simulink model "Multiagent_1030_ActorCritic"  (R2023a)
settings: Solver=FixedStepAuto  StartTime=0.0  StopTime=500  FixedStep=0.001  RelTol=1e-3
values from neighbouring files (symbols this model uses):
  INT_1 = [0;0.5;0]    [Paramaters.m]
  INT_2 = [-3.5;6;0]    [Paramaters.m]
  INT_3 = [-7.1;10;0.0]    [Paramaters.m]
  INT_4 = [-10.5;15;0.2]    [Paramaters.m]
  INT_5 = [-14;20;0.4]    [Paramaters.m]
(part 1 of 2)
settings Model: Creator=Admin  LastModifiedBy=ADMIN
settings DataIOCC: ReturnWorkspaceOutputs=off
settings DebuggingCC: UnconnectedInputMsg=warning  UnconnectedOutputMsg=warning  UnconnectedLineMsg=warning
settings ModelReferenceCC: EnableRefExpFcnMdlSchedulingChecks=on
settings RTWCC: DLArmComputeVersion=19.05

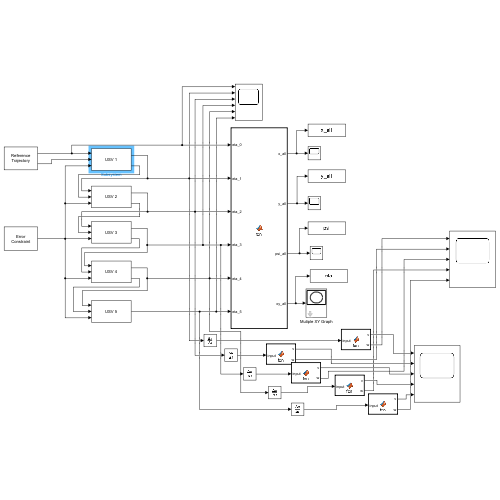
[thumbnail: Simulink's stored preview of the top-level diagram]
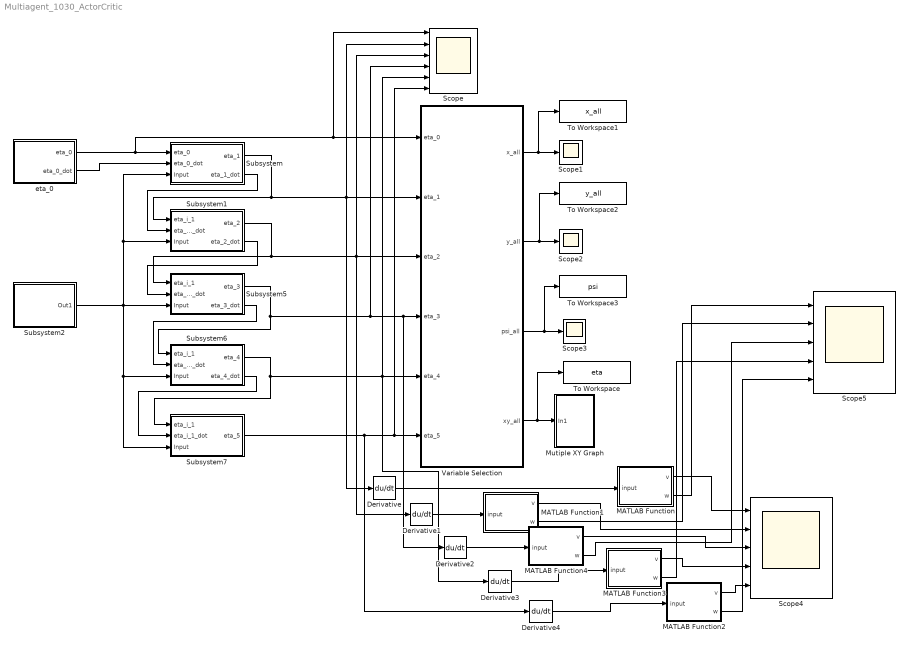
== system Multiagent_1030_ActorCritic ==
  Derivative{,1..4} (5 alike) : Derivative
  MATLAB Function : MATLAB Function  TreatAsAtomicUnit=on
  MATLAB Function1 : MATLAB Function  TreatAsAtomicUnit=on
  MATLAB Function2 : MATLAB Function  TreatAsAtomicUnit=on
  MATLAB Function3 : MATLAB Function  TreatAsAtomicUnit=on
  MATLAB Function4 : MATLAB Function  TreatAsAtomicUnit=on
  Mutiple XY Graph : Subsystem  mask(Mutiple XY Graph){number_of_trajectories=5, axis_limits=[-40 80 -10 110], sample_time=1}
      mask prompts: number_of_trajectories "Number of Trajectories"; axis_limits "Axis Limits"; sample_time "Sample Time"
      mask Display: plot([.05 .95 .95 .05 .05],[.45 .45 .95 .95 .45], 0.5+cos(0:0.1:2*pi)*0.3,0.7+sin(0:0.1:2*pi)*0.2)
  Scope : Scope  NumInputPorts=6
  Scope1 : Scope
  Scope2 : Scope
  Scope3 : Scope
  Scope4 : Scope  NumInputPorts=5
  Scope5 : Scope  NumInputPorts=5
  Subsystem : Subsystem
      mask Display: disp('USV 1')
  Subsystem1 : Subsystem
      mask Display: disp('USV 2')
  Subsystem2 : Subsystem
      mask Display: disp('Error\nConstraint');
  Subsystem5 : Subsystem
      mask Display: disp('USV 3')
  Subsystem6 : Subsystem
      mask Display: disp('USV 4')
  Subsystem7 : Subsystem
      mask Display: disp('USV 5')
  To Workspace : ToWorkspace  VariableName=eta  SaveFormat=Timeseries  SampleTime=-1
  To Workspace1 : ToWorkspace  VariableName=x_all  SaveFormat=Timeseries  SampleTime=-1
  To Workspace2 : ToWorkspace  VariableName=y_all  SaveFormat=Timeseries  SampleTime=-1
  To Workspace3 : ToWorkspace  VariableName=psi  SaveFormat=Timeseries  SampleTime=-1
  Variable Selection : MATLAB Function  TreatAsAtomicUnit=on
  eta_0 : Subsystem
      mask Display: disp('Reference\nTrajectory')
  wires:
  Subsystem/1(eta_1) -> Subsystem1/1(eta_i_1), Scope/2, Variable Selection/2(eta_1), Derivative/1
  Variable Selection/4(xy_all) -> To Workspace/1, Mutiple XY Graph/1(In1)
  eta_0/1(eta_0) -> Scope/1, Variable Selection/1(eta_0), Subsystem/1(eta_0)
  eta_0/2(eta_0_dot) -> Subsystem/2(eta_0_dot)
  Subsystem/2(eta_1_dot) -> Subsystem1/2(eta_i_1_dot)
  Subsystem1/1(eta_2) -> Variable Selection/3(eta_2), Scope/3, Derivative1/1, Subsystem5/1(eta_i_1)
  Variable Selection/1(x_all) -> To Workspace1/1, Scope1/1
  Variable Selection/2(y_all) -> To Workspace2/1, Scope2/1
  Variable Selection/3(psi_all) -> To Workspace3/1, Scope3/1
  Subsystem7/1(eta_5) -> Variable Selection/6(eta_5), Scope/6, Derivative4/1
  Subsystem6/1(eta_4) -> Subsystem7/1(eta_i_1), Scope/5, Variable Selection/5(eta_4), Derivative3/1
  Subsystem6/2(eta_4_dot) -> Subsystem7/2(eta_i_1_dot)
  Subsystem5/1(eta_3) -> Variable Selection/4(eta_3), Derivative2/1, Scope/4, Subsystem6/1(eta_i_1)
  Subsystem5/2(eta_3_dot) -> Subsystem6/2(eta_i_1_dot)
  Subsystem1/2(eta_2_dot) -> Subsystem5/2(eta_i_1_dot)
  Subsystem2/1(Out1) -> Subsystem1/3(Input), Subsystem/3(Input), Subsystem7/3(Input), Subsystem6/3(Input), Subsystem5/3(Input)
  Derivative/1 -> MATLAB Function/1(input)
  MATLAB Function/1(v) -> Scope4/1
  Derivative1/1 -> MATLAB Function1/1(input)
  Derivative2/1 -> MATLAB Function4/1(input)
  Derivative3/1 -> MATLAB Function3/1(input)
  Derivative4/1 -> MATLAB Function2/1(input)
  MATLAB Function1/1(v) -> Scope4/2
  MATLAB Function4/1(v) -> Scope4/3
  MATLAB Function3/1(v) -> Scope4/4
  MATLAB Function2/1(v) -> Scope4/5
  MATLAB Function/2(w) -> Scope5/1
  MATLAB Function1/2(w) -> Scope5/2
  MATLAB Function4/2(w) -> Scope5/3
  MATLAB Function3/2(w) -> Scope5/4
  MATLAB Function2/2(w) -> Scope5/5

== system Multiagent_1030_ActorCritic/Mutiple XY Graph ==
  In1 : Inport
  Level-2 MATLAB S-Function : M-S-Function  FunctionName=multiple_xy_graph  Parameters=number_of_trajectories,axis_limits
  Rate Transition : RateTransition  OutPortSampleTime=sample_time
  wires:
  In1/1 -> Rate Transition/1
  Rate Transition/1 -> Level-2 MATLAB S-Function/1

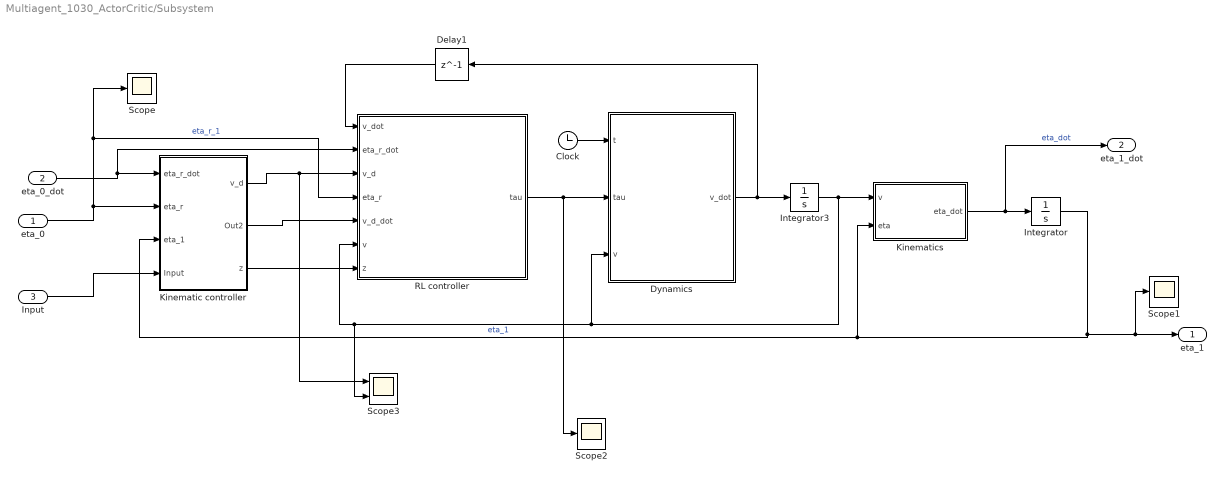
== system Multiagent_1030_ActorCritic/Subsystem ==
  eta_0 : Inport
  eta_0_dot : Inport  Port=2
  Input : Inport  Port=3
  Clock : Clock
  Delay1 : Delay  DelayLength=1  InitialCondition=[0;0;0]  SampleTime=0.001
  Dynamics : MATLAB Function  TreatAsAtomicUnit=on
  Integrator : Integrator  InitialCondition=INT_1
  Integrator3 : Integrator  InitialCondition=[0;0;0]
  Kinematic controller : Subsystem
  Kinematics : MATLAB Function  TreatAsAtomicUnit=on
  RL controller : Subsystem
  Scope : Scope
  Scope1 : Scope
  Scope2 : Scope
  Scope3 : Scope  NumInputPorts=2
  eta_1 : Outport
  eta_1_dot : Outport  Port=2
  wires:
  Kinematics/1(eta_dot) -> Integrator/1, eta_1_dot/1  "eta_dot"
  Integrator/1 -> Kinematics/2(eta), Kinematic controller/3(eta_1), Scope1/1, eta_1/1  "eta_1"
  eta_0/1 -> RL controller/4(eta_r), Scope/1, Kinematic controller/2(eta_r)  "eta_r_1"
  Dynamics/1(v_dot) -> Integrator3/1, Delay1/1
  Integrator3/1 -> Dynamics/3(v), Scope3/2, RL controller/6(v), Kinematics/1(v)
  eta_0_dot/1 -> RL controller/2(eta_r_dot), Kinematic controller/1(eta_r_dot)
  Delay1/1 -> RL controller/1(v_dot)
  Kinematic controller/1(v_d) -> RL controller/3(v_d), Scope3/1
  Kinematic controller/2(Out2) -> RL controller/5(v_d_dot)
  Kinematic controller/3(z) -> RL controller/7(z)
  Clock/1 -> Dynamics/1(t)
  Input/1 -> Kinematic controller/4(Input)
  RL controller/1(tau) -> Scope2/1, Dynamics/2(tau)

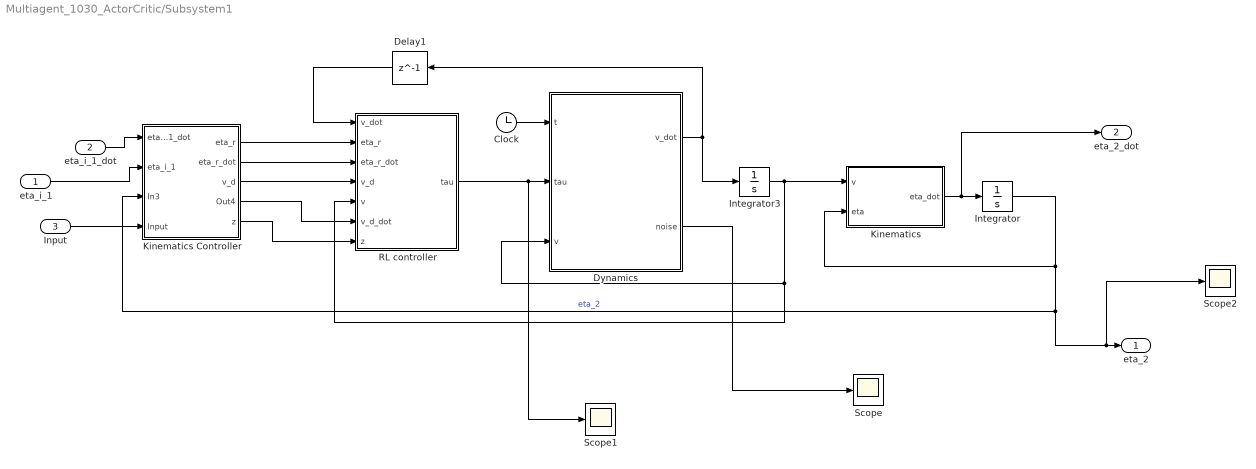
== system Multiagent_1030_ActorCritic/Subsystem1 ==
  eta_i_1 : Inport
  eta_i_1_dot : Inport  Port=2
  Input : Inport  Port=3
  Clock : Clock
  Delay1 : Delay  DelayLength=1  InitialCondition=[0;0;0]  SampleTime=0.001
  Dynamics : MATLAB Function  TreatAsAtomicUnit=on
  Integrator : Integrator  InitialCondition=INT_2
  Integrator3 : Integrator  InitialCondition=[0;0;0]
  Kinematics : MATLAB Function  TreatAsAtomicUnit=on
  Kinematics Controller : Subsystem
  RL controller : Subsystem
  Scope : Scope
  Scope1 : Scope
  Scope2 : Scope
  eta_2 : Outport
  eta_2_dot : Outport  Port=2
  wires:
  Integrator3/1 -> Dynamics/3(v), RL controller/5(v), Kinematics/1(v)
  Dynamics/1(v_dot) -> Integrator3/1, Delay1/1
  Clock/1 -> Dynamics/1(t)
  Integrator/1 -> Scope2/1, eta_2/1, Kinematics Controller/3(In3), Kinematics/2(eta)  "eta_2"
  Kinematics/1(eta_dot) -> eta_2_dot/1, Integrator/1
  eta_i_1_dot/1 -> Kinematics Controller/1(eta_i_1_dot)
  eta_i_1/1 -> Kinematics Controller/2(eta_i_1)
  Delay1/1 -> RL controller/1(v_dot)
  Kinematics Controller/1(eta_r) -> RL controller/2(eta_r)
  Kinematics Controller/2(eta_r_dot) -> RL controller/3(eta_r_dot)
  Kinematics Controller/3(v_d) -> RL controller/4(v_d)
  Kinematics Controller/4(Out4) -> RL controller/6(v_d_dot)
  Kinematics Controller/5(z) -> RL controller/7(z)
  Dynamics/2(noise) -> Scope/1
  Input/1 -> Kinematics Controller/4(Input)
  RL controller/1(tau) -> Scope1/1, Dynamics/2(tau)

== system Multiagent_1030_ActorCritic/Subsystem2 ==
  Clock2 : Clock
  MATLAB Function2 : MATLAB Function  TreatAsAtomicUnit=on
  Mux : Mux  Inputs=6
  To Workspace : ToWorkspace  VariableName=e1  SampleTime=-1
      settings: Save2DSignal=2-D array (concatenate along first dimension)
  To Workspace1 : ToWorkspace  VariableName=e2  SampleTime=-1
      settings: Save2DSignal=2-D array (concatenate along first dimension)
  Out1 : Outport
  wires:
  Clock2/1 -> MATLAB Function2/1(t)
  MATLAB Function2/1(e1) -> To Workspace/1, To Workspace1/1, Mux/1
  MATLAB Function2/2(e2) -> Mux/2
  MATLAB Function2/3(e1_dot) -> Mux/3
  MATLAB Function2/4(e2_dot) -> Mux/4
  MATLAB Function2/5(gamma) -> Mux/5
  MATLAB Function2/6(gamma_dot) -> Mux/6
  Mux/1 -> Out1/1

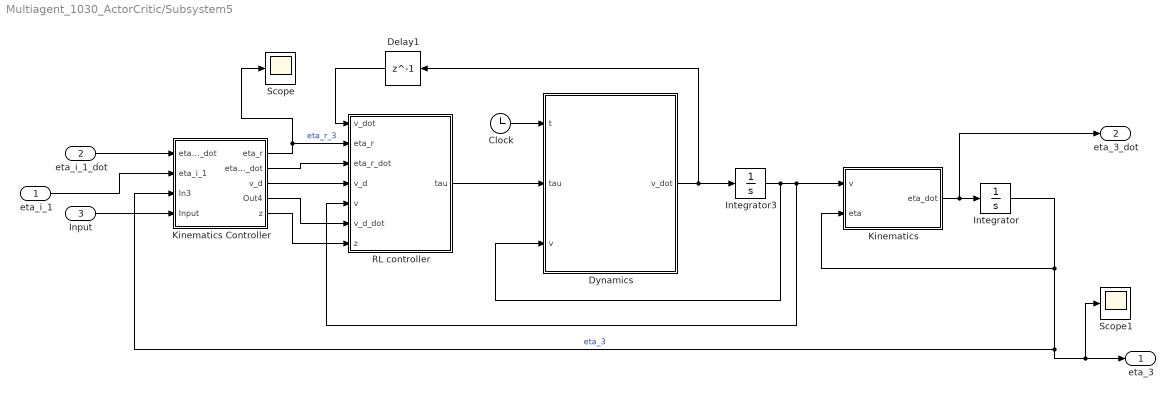
== system Multiagent_1030_ActorCritic/Subsystem5 ==
  eta_i_1 : Inport
  eta_i_1_dot : Inport  Port=2
  Input : Inport  Port=3
  Clock : Clock
  Delay1 : Delay  DelayLength=1  InitialCondition=[0;0;0]  SampleTime=0.001
  Dynamics : MATLAB Function  TreatAsAtomicUnit=on
  Integrator : Integrator  InitialCondition=INT_3
  Integrator3 : Integrator  InitialCondition=[0;0;0]
  Kinematics : MATLAB Function  TreatAsAtomicUnit=on
  Kinematics Controller : Subsystem
  RL controller : Subsystem
  Scope : Scope
  Scope1 : Scope
  eta_3 : Outport
  eta_3_dot : Outport  Port=2
  wires:
  Kinematics Controller/5(z) -> RL controller/7(z)
  Kinematics Controller/4(Out4) -> RL controller/6(v_d_dot)
  Kinematics Controller/3(v_d) -> RL controller/4(v_d)
  Kinematics Controller/2(eta_r_dot) -> RL controller/3(eta_r_dot)
  Kinematics Controller/1(eta_r) -> Scope/1, RL controller/2(eta_r)  "eta_r_3"
  Delay1/1 -> RL controller/1(v_dot)
  eta_i_1/1 -> Kinematics Controller/2(eta_i_1)
  eta_i_1_dot/1 -> Kinematics Controller/1(eta_i_1_dot)
  Kinematics/1(eta_dot) -> Integrator/1, eta_3_dot/1
  Integrator/1 -> Kinematics/2(eta), Scope1/1, eta_3/1, Kinematics Controller/3(In3)  "eta_3"
  Clock/1 -> Dynamics/1(t)
  Dynamics/1(v_dot) -> Integrator3/1, Delay1/1
  Integrator3/1 -> RL controller/5(v), Kinematics/1(v), Dynamics/3(v)
  Input/1 -> Kinematics Controller/4(Input)
  RL controller/1(tau) -> Dynamics/2(tau)

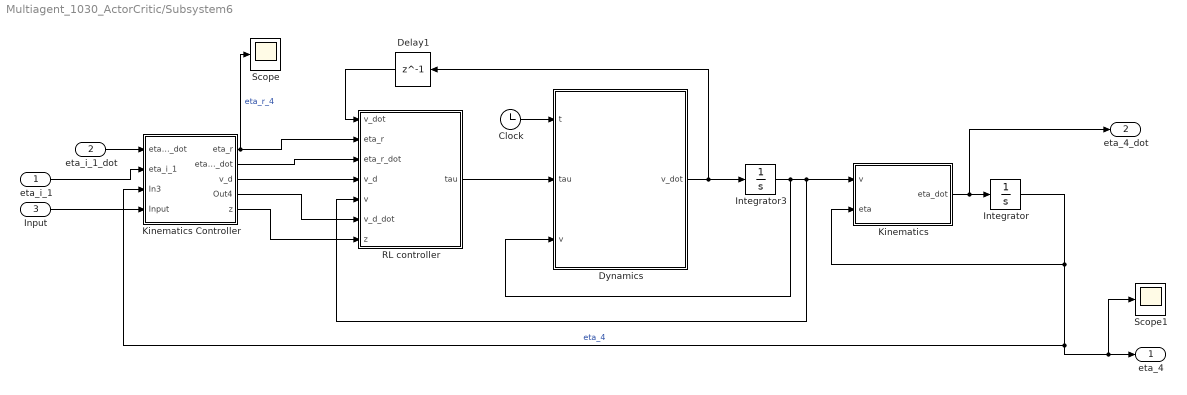
== system Multiagent_1030_ActorCritic/Subsystem6 ==
  eta_i_1 : Inport
  eta_i_1_dot : Inport  Port=2
  Input : Inport  Port=3
  Clock : Clock
  Delay1 : Delay  DelayLength=1  InitialCondition=[0;0;0]  SampleTime=0.001
  Dynamics : MATLAB Function  TreatAsAtomicUnit=on
  Integrator : Integrator  InitialCondition=INT_4
  Integrator3 : Integrator  InitialCondition=[0;0;0]
  Kinematics : MATLAB Function  TreatAsAtomicUnit=on
  Kinematics Controller : Subsystem
  RL controller : Subsystem
  Scope : Scope
  Scope1 : Scope
  eta_4 : Outport
  eta_4_dot : Outport  Port=2
  wires:
  Integrator3/1 -> Dynamics/3(v), Kinematics/1(v), RL controller/5(v)
  Dynamics/1(v_dot) -> Delay1/1, Integrator3/1
  Clock/1 -> Dynamics/1(t)
  Integrator/1 -> Scope1/1, eta_4/1, Kinematics Controller/3(In3), Kinematics/2(eta)  "eta_4"
  Kinematics/1(eta_dot) -> eta_4_dot/1, Integrator/1
  eta_i_1_dot/1 -> Kinematics Controller/1(eta_i_1_dot)
  eta_i_1/1 -> Kinematics Controller/2(eta_i_1)
  Delay1/1 -> RL controller/1(v_dot)
  Kinematics Controller/1(eta_r) -> Scope/1, RL controller/2(eta_r)  "eta_r_4"
  Kinematics Controller/2(eta_r_dot) -> RL controller/3(eta_r_dot)
  Kinematics Controller/3(v_d) -> RL controller/4(v_d)
  Kinematics Controller/4(Out4) -> RL controller/6(v_d_dot)
  Kinematics Controller/5(z) -> RL controller/7(z)
  Input/1 -> Kinematics Controller/4(Input)
  RL controller/1(tau) -> Dynamics/2(tau)

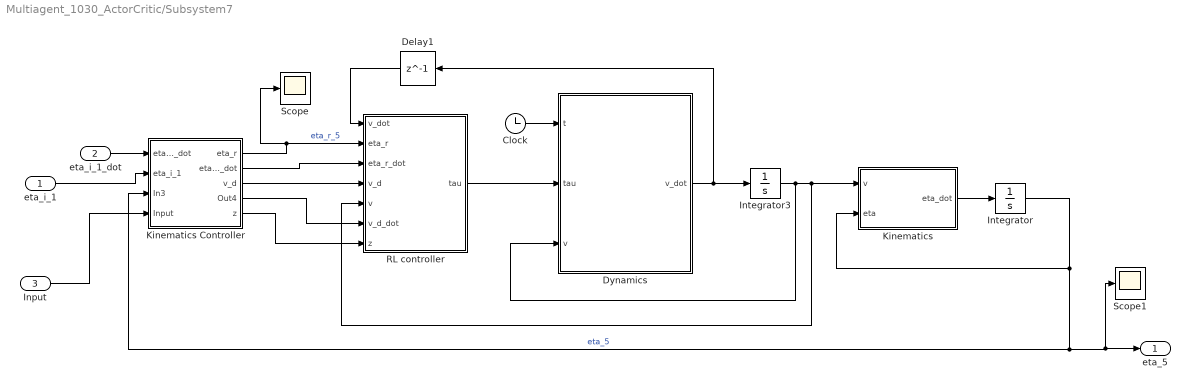
== system Multiagent_1030_ActorCritic/Subsystem7 ==
  eta_i_1 : Inport
  eta_i_1_dot : Inport  Port=2
  Input : Inport  Port=3
  Clock : Clock
  Delay1 : Delay  DelayLength=1  InitialCondition=[0;0;0]  SampleTime=0.001
  Dynamics : MATLAB Function  TreatAsAtomicUnit=on
  Integrator : Integrator  InitialCondition=INT_5
  Integrator3 : Integrator  InitialCondition=[0;0;0]
  Kinematics : MATLAB Function  TreatAsAtomicUnit=on
  Kinematics Controller : Subsystem
  RL controller : Subsystem
  Scope : Scope
  Scope1 : Scope
  eta_5 : Outport
  wires:
  Kinematics Controller/5(z) -> RL controller/7(z)
  Kinematics Controller/4(Out4) -> RL controller/6(v_d_dot)
  Kinematics Controller/3(v_d) -> RL controller/4(v_d)
  Kinematics Controller/2(eta_r_dot) -> RL controller/3(eta_r_dot)
  Kinematics Controller/1(eta_r) -> Scope/1, RL controller/2(eta_r)  "eta_r_5"
  Delay1/1 -> RL controller/1(v_dot)
  eta_i_1/1 -> Kinematics Controller/2(eta_i_1)
  eta_i_1_dot/1 -> Kinematics Controller/1(eta_i_1_dot)
  Kinematics/1(eta_dot) -> Integrator/1
  Integrator/1 -> Kinematics/2(eta), Scope1/1, eta_5/1, Kinematics Controller/3(In3)  "eta_5"
  Clock/1 -> Dynamics/1(t)
  Dynamics/1(v_dot) -> Integrator3/1, Delay1/1
  Integrator3/1 -> RL controller/5(v), Kinematics/1(v), Dynamics/3(v)
  Input/1 -> Kinematics Controller/4(Input)
  RL controller/1(tau) -> Dynamics/2(tau)

== system Multiagent_1030_ActorCritic/eta_0 ==
  Clock1 : Clock
  MATLAB Function : MATLAB Function  TreatAsAtomicUnit=on
  eta_0 : Outport
  eta_0_dot : Outport  Port=2
  wires:
  Clock1/1 -> MATLAB Function/1(t)
  MATLAB Function/1(eta_r) -> eta_0/1
  MATLAB Function/2(eta_r_dot) -> eta_0_dot/1

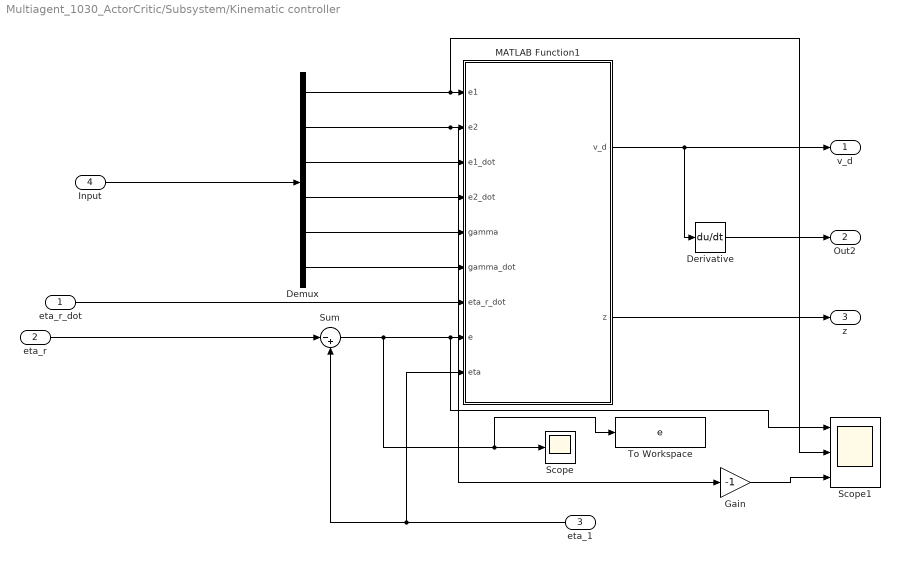
== system Multiagent_1030_ActorCritic/Subsystem/Kinematic controller ==
  eta_r_dot : Inport
  eta_r : Inport  Port=2
  eta_1 : Inport  Port=3
  Input : Inport  Port=4
  Demux : Demux  Outputs=6
  Derivative : Derivative
  Gain : Gain  Gain=-1
  MATLAB Function1 : MATLAB Function  TreatAsAtomicUnit=on
  Scope : Scope
  Scope1 : Scope  NumInputPorts=3
  Sum : Sum  Inputs=|-+
  To Workspace : ToWorkspace  VariableName=e  SampleTime=-1
      settings: Save2DSignal=2-D array (concatenate along first dimension)
  v_d : Outport
  Out2 : Outport  Port=2
  z : Outport  Port=3
  wires:
  MATLAB Function1/1(v_d) -> Derivative/1, v_d/1
  Sum/1 -> To Workspace/1, Scope/1, Scope1/1, MATLAB Function1/8(e)
  eta_r/1 -> Sum/1
  eta_1/1 -> MATLAB Function1/9(eta), Sum/2
  eta_r_dot/1 -> MATLAB Function1/7(eta_r_dot)
  Derivative/1 -> Out2/1
  MATLAB Function1/2(z) -> z/1
  Demux/1 -> Scope1/2, MATLAB Function1/1(e1)
  Demux/2 -> Gain/1, MATLAB Function1/2(e2)
  Demux/3 -> MATLAB Function1/3(e1_dot)
  Demux/4 -> MATLAB Function1/4(e2_dot)
  Demux/5 -> MATLAB Function1/5(gamma)
  Demux/6 -> MATLAB Function1/6(gamma_dot)
  Input/1 -> Demux/1
  Gain/1 -> Scope1/3

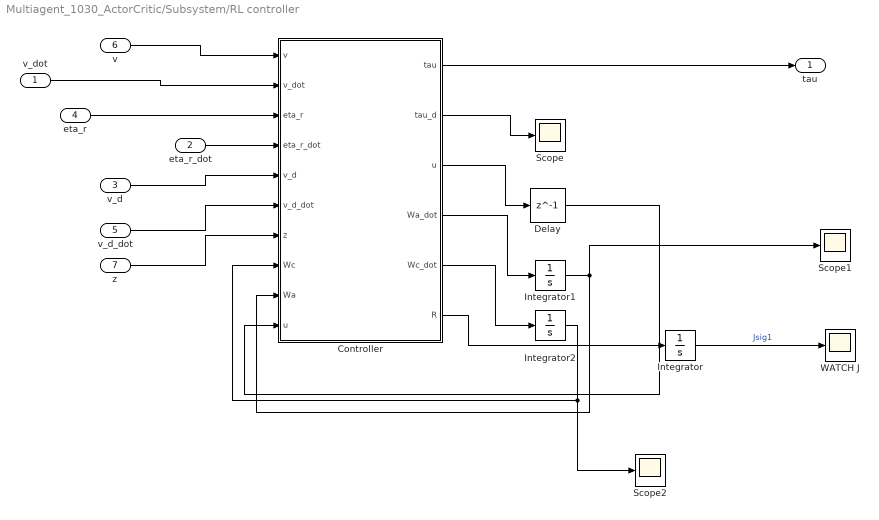
== system Multiagent_1030_ActorCritic/Subsystem/RL controller ==
  v_dot : Inport
  eta_r_dot : Inport  Port=2
  v_d : Inport  Port=3
  eta_r : Inport  Port=4
  v_d_dot : Inport  Port=5
  v : Inport  Port=6
  z : Inport  Port=7
  Controller : MATLAB Function  TreatAsAtomicUnit=on
  Delay : Delay  DelayLength=1  InitialCondition=[0;0;0]  SampleTime=0.001
  Integrator : Integrator
  Integrator1 : Integrator  InitialCondition=zeros(15,1)
  Integrator2 : Integrator  InitialCondition=zeros(15,1)
  Scope : Scope
  Scope1 : Scope
  Scope2 : Scope
  WATCH J : Scope
  tau : Outport
  wires:
  Delay/1 -> Controller/10("u ")
  Controller/2(tau_d) -> Scope/1
  Controller/1(tau) -> tau/1
  Integrator1/1 -> Scope1/1, Controller/9(Wa)
  Controller/4(Wa_dot) -> Integrator1/1
  v_d/1 -> Controller/5(v_d)
  Controller/3(u) -> Delay/1
  Controller/5(Wc_dot) -> Integrator2/1
  Integrator2/1 -> Scope2/1, Controller/8(Wc)
  v_d_dot/1 -> Controller/6(v_d_dot)
  z/1 -> Controller/7(z)
  v/1 -> Controller/1(v)
  v_dot/1 -> Controller/2(v_dot)
  eta_r_dot/1 -> Controller/4(eta_r_dot)
  eta_r/1 -> Controller/3(eta_r)
  Controller/6(R) -> Integrator/1
  Integrator/1 -> WATCH J/1  "Jsig1"

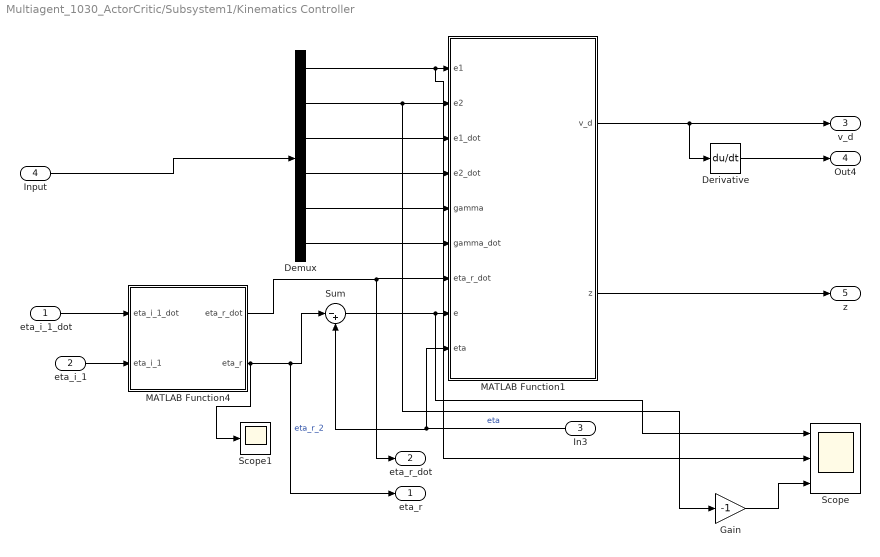
== system Multiagent_1030_ActorCritic/Subsystem1/Kinematics Controller ==
  eta_i_1_dot : Inport
  eta_i_1 : Inport  Port=2
  In3 : Inport  Port=3
  Input : Inport  Port=4
  Demux : Demux  Outputs=6
  Derivative : Derivative
  Gain : Gain  Gain=-1
  MATLAB Function1 : MATLAB Function  TreatAsAtomicUnit=on
  MATLAB Function4 : MATLAB Function  TreatAsAtomicUnit=on
  Scope : Scope  NumInputPorts=3
  Scope1 : Scope
  Sum : Sum  Inputs=|-+
  eta_r : Outport
  eta_r_dot : Outport  Port=2
  v_d : Outport  Port=3
  Out4 : Outport  Port=4
  z : Outport  Port=5
  wires:
  MATLAB Function1/1(v_d) -> Derivative/1, v_d/1
  Sum/1 -> Scope/1, MATLAB Function1/8(e)
  MATLAB Function4/2(eta_r) -> Scope1/1, eta_r/1, Sum/1  "eta_r_2"
  MATLAB Function1/2(z) -> z/1
  eta_i_1_dot/1 -> MATLAB Function4/1(eta_i_1_dot)
  MATLAB Function4/1(eta_r_dot) -> MATLAB Function1/7(eta_r_dot), eta_r_dot/1
  In3/1 -> Sum/2, MATLAB Function1/9(eta)  "eta"
  eta_i_1/1 -> MATLAB Function4/2(eta_i_1)
  Derivative/1 -> Out4/1
  Demux/1 -> Scope/2, MATLAB Function1/1(e1)
  Demux/2 -> MATLAB Function1/2(e2), Gain/1
  Demux/3 -> MATLAB Function1/3(e1_dot)
  Demux/4 -> MATLAB Function1/4(e2_dot)
  Demux/5 -> MATLAB Function1/5(gamma)
  Demux/6 -> MATLAB Function1/6(gamma_dot)
  Input/1 -> Demux/1
  Gain/1 -> Scope/3

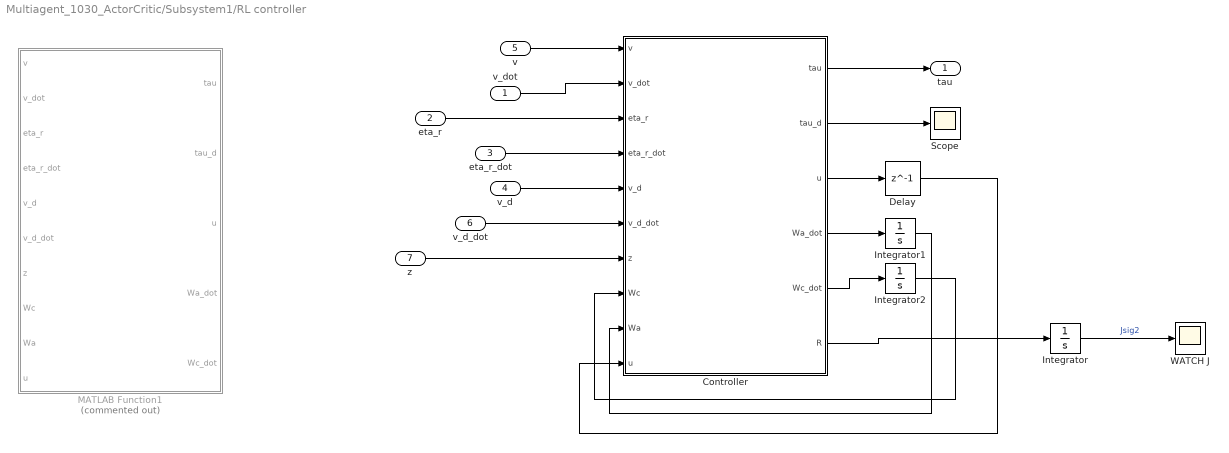
== system Multiagent_1030_ActorCritic/Subsystem1/RL controller ==
  v_dot : Inport
  eta_r : Inport  Port=2
  eta_r_dot : Inport  Port=3
  v_d : Inport  Port=4
  v : Inport  Port=5
  v_d_dot : Inport  Port=6
  z : Inport  Port=7
  Controller : MATLAB Function  TreatAsAtomicUnit=on
  Delay : Delay  DelayLength=1  InitialCondition=[0;0;0]  SampleTime=0.001
  Integrator : Integrator
  Integrator1 : Integrator  InitialCondition=zeros(15,1)
  Integrator2 : Integrator  InitialCondition=zeros(15,1)
  MATLAB Function1 : MATLAB Function  Commented=on  TreatAsAtomicUnit=on
  Scope : Scope
  WATCH J : Scope
  tau : Outport
  wires:
  Delay/1 -> Controller/10("u ")
  v_dot/1 -> Controller/2(v_dot)
  Controller/3(u) -> Delay/1
  Controller/4(Wa_dot) -> Integrator1/1
  Controller/2(tau_d) -> Scope/1
  Controller/5(Wc_dot) -> Integrator2/1
  Integrator2/1 -> Controller/8(Wc)
  eta_r/1 -> Controller/3(eta_r)
  Integrator1/1 -> Controller/9(Wa)
  eta_r_dot/1 -> Controller/4(eta_r_dot)
  v_d/1 -> Controller/5(v_d)
  v_d_dot/1 -> Controller/6(v_d_dot)
  z/1 -> Controller/7(z)
  Controller/1(tau) -> tau/1
  v/1 -> Controller/1(v)
  Controller/6(R) -> Integrator/1
  Integrator/1 -> WATCH J/1  "Jsig2"

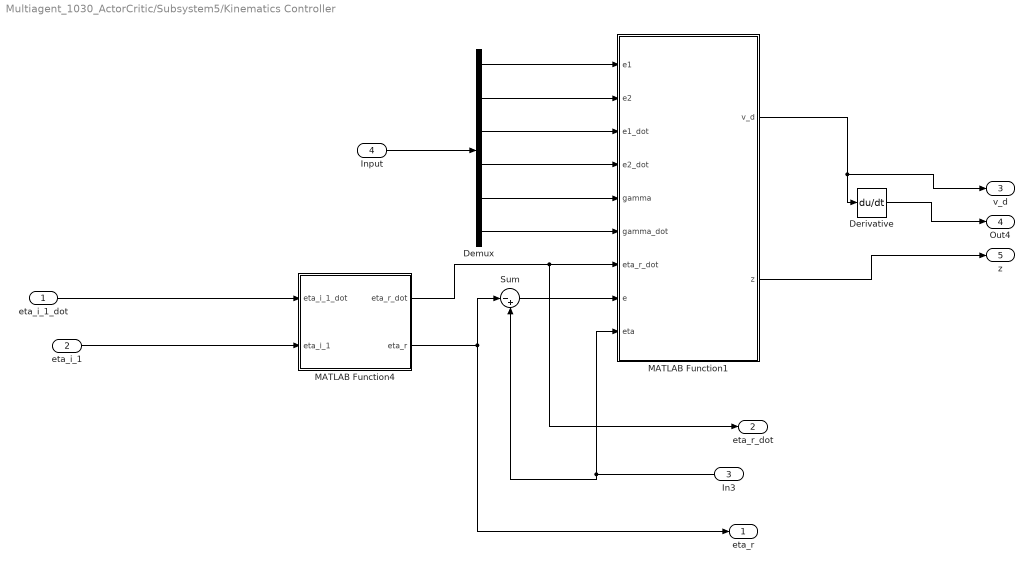
== system Multiagent_1030_ActorCritic/Subsystem5/Kinematics Controller ==
  eta_i_1_dot : Inport
  eta_i_1 : Inport  Port=2
  In3 : Inport  Port=3
  Input : Inport  Port=4
  Demux : Demux  Outputs=6
  Derivative : Derivative
  MATLAB Function1 : MATLAB Function  TreatAsAtomicUnit=on
  MATLAB Function4 : MATLAB Function  TreatAsAtomicUnit=on
  Sum : Sum  Inputs=|-+
  eta_r : Outport
  eta_r_dot : Outport  Port=2
  v_d : Outport  Port=3
  Out4 : Outport  Port=4
  z : Outport  Port=5
  wires:
  Derivative/1 -> Out4/1
  eta_i_1/1 -> MATLAB Function4/2(eta_i_1)
  In3/1 -> Sum/2, MATLAB Function1/9(eta)
  MATLAB Function4/1(eta_r_dot) -> MATLAB Function1/7(eta_r_dot), eta_r_dot/1
  eta_i_1_dot/1 -> MATLAB Function4/1(eta_i_1_dot)
  MATLAB Function1/2(z) -> z/1
  MATLAB Function4/2(eta_r) -> Sum/1, eta_r/1
  Sum/1 -> MATLAB Function1/8(e)
  MATLAB Function1/1(v_d) -> Derivative/1, v_d/1
  Input/1 -> Demux/1
  Demux/1 -> MATLAB Function1/1(e1)
  Demux/2 -> MATLAB Function1/2(e2)
  Demux/3 -> MATLAB Function1/3(e1_dot)
  Demux/4 -> MATLAB Function1/4(e2_dot)
  Demux/5 -> MATLAB Function1/5(gamma)
  Demux/6 -> MATLAB Function1/6(gamma_dot)

== system Multiagent_1030_ActorCritic/Subsystem5/RL controller ==
  v_dot : Inport
  eta_r : Inport  Port=2
  eta_r_dot : Inport  Port=3
  v_d : Inport  Port=4
  v : Inport  Port=5
  v_d_dot : Inport  Port=6
  z : Inport  Port=7
  Delay : Delay  DelayLength=1  InitialCondition=[0;0;0]  SampleTime=0.001
  Integrator1 : Integrator  InitialCondition=zeros(15,1)
  Integrator2 : Integrator  InitialCondition=zeros(15,1)
  MATLAB Function : MATLAB Function  TreatAsAtomicUnit=on
  Scope : Scope
  tau : Outport
  wires:
  v/1 -> MATLAB Function/1(v)
  MATLAB Function/1(tau) -> tau/1
  z/1 -> MATLAB Function/7(z)
  v_d_dot/1 -> MATLAB Function/6(v_d_dot)
  v_d/1 -> MATLAB Function/5(v_d)
  eta_r_dot/1 -> MATLAB Function/4(eta_r_dot)
  Integrator1/1 -> MATLAB Function/9(Wa)
  eta_r/1 -> MATLAB Function/3(eta_r)
  Integrator2/1 -> MATLAB Function/8(Wc)
  MATLAB Function/5(Wc_dot) -> Integrator2/1
  MATLAB Function/2(tau_d) -> Scope/1
  MATLAB Function/4(Wa_dot) -> Integrator1/1
  MATLAB Function/3(u) -> Delay/1
  v_dot/1 -> MATLAB Function/2(v_dot)
  Delay/1 -> MATLAB Function/10("u ")

== system Multiagent_1030_ActorCritic/Subsystem6/Kinematics Controller ==
  eta_i_1_dot : Inport
  eta_i_1 : Inport  Port=2
  In3 : Inport  Port=3
  Input : Inport  Port=4
  Demux : Demux  Outputs=6
  Derivative : Derivative
  MATLAB Function1 : MATLAB Function  TreatAsAtomicUnit=on
  MATLAB Function4 : MATLAB Function  TreatAsAtomicUnit=on
  Sum : Sum  Inputs=|-+
  eta_r : Outport
  eta_r_dot : Outport  Port=2
  v_d : Outport  Port=3
  Out4 : Outport  Port=4
  z : Outport  Port=5
  wires:
  MATLAB Function1/1(v_d) -> v_d/1, Derivative/1
  Sum/1 -> MATLAB Function1/8(e)
  MATLAB Function4/2(eta_r) -> eta_r/1, Sum/1
  MATLAB Function1/2(z) -> z/1
  eta_i_1_dot/1 -> MATLAB Function4/1(eta_i_1_dot)
  MATLAB Function4/1(eta_r_dot) -> eta_r_dot/1, MATLAB Function1/7(eta_r_dot)
  In3/1 -> Sum/2, MATLAB Function1/9(eta)
  eta_i_1/1 -> MATLAB Function4/2(eta_i_1)
  Derivative/1 -> Out4/1
  Demux/6 -> MATLAB Function1/6(gamma_dot)
  Demux/5 -> MATLAB Function1/5(gamma)
  Demux/4 -> MATLAB Function1/4(e2_dot)
  Demux/3 -> MATLAB Function1/3(e1_dot)
  Demux/2 -> MATLAB Function1/2(e2)
  Demux/1 -> MATLAB Function1/1(e1)
  Input/1 -> Demux/1

== system Multiagent_1030_ActorCritic/Subsystem6/RL controller ==
  v_dot : Inport
  eta_r : Inport  Port=2
  eta_r_dot : Inport  Port=3
  v_d : Inport  Port=4
  v : Inport  Port=5
  v_d_dot : Inport  Port=6
  z : Inport  Port=7
  Delay : Delay  DelayLength=1  InitialCondition=[0;0;0]  SampleTime=0.001
  Integrator1 : Integrator  InitialCondition=zeros(15,1)
  Integrator2 : Integrator  InitialCondition=zeros(15,1)
  MATLAB Function : MATLAB Function  TreatAsAtomicUnit=on
  Scope : Scope
  tau : Outport
  wires:
  Delay/1 -> MATLAB Function/10("u ")
  v_dot/1 -> MATLAB Function/2(v_dot)
  MATLAB Function/3(u) -> Delay/1
  MATLAB Function/4(Wa_dot) -> Integrator1/1
  MATLAB Function/2(tau_d) -> Scope/1
  MATLAB Function/5(Wc_dot) -> Integrator2/1
  Integrator2/1 -> MATLAB Function/8(Wc)
  eta_r/1 -> MATLAB Function/3(eta_r)
  Integrator1/1 -> MATLAB Function/9(Wa)
  eta_r_dot/1 -> MATLAB Function/4(eta_r_dot)
  v_d/1 -> MATLAB Function/5(v_d)
  v_d_dot/1 -> MATLAB Function/6(v_d_dot)
  z/1 -> MATLAB Function/7(z)
  MATLAB Function/1(tau) -> tau/1
  v/1 -> MATLAB Function/1(v)

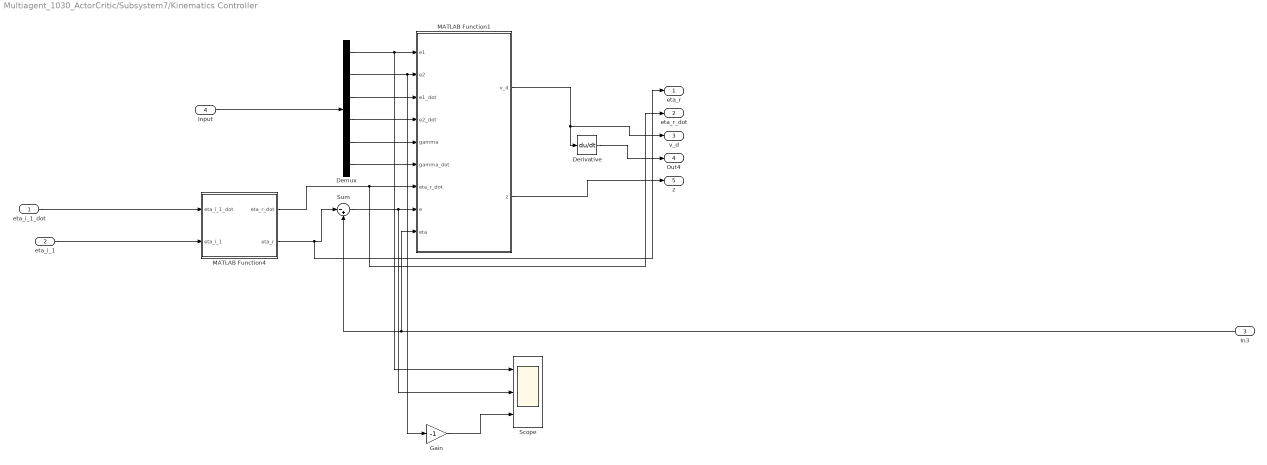
== system Multiagent_1030_ActorCritic/Subsystem7/Kinematics Controller ==
  eta_i_1_dot : Inport
  eta_i_1 : Inport  Port=2
  In3 : Inport  Port=3
  Input : Inport  Port=4
  Demux : Demux  Outputs=6
  Derivative : Derivative
  Gain : Gain  Gain=-1
  MATLAB Function1 : MATLAB Function  TreatAsAtomicUnit=on
  MATLAB Function4 : MATLAB Function  TreatAsAtomicUnit=on
  Scope : Scope  NumInputPorts=3
  Sum : Sum  Inputs=|-+
  eta_r : Outport
  eta_r_dot : Outport  Port=2
  v_d : Outport  Port=3
  Out4 : Outport  Port=4
  z : Outport  Port=5
  wires:
  Derivative/1 -> Out4/1
  eta_i_1/1 -> MATLAB Function4/2(eta_i_1)
  In3/1 -> MATLAB Function1/9(eta), Sum/2
  MATLAB Function4/1(eta_r_dot) -> MATLAB Function1/7(eta_r_dot), eta_r_dot/1
  eta_i_1_dot/1 -> MATLAB Function4/1(eta_i_1_dot)
  MATLAB Function1/2(z) -> z/1
  MATLAB Function4/2(eta_r) -> Sum/1, eta_r/1
  Sum/1 -> Scope/2, MATLAB Function1/8(e)
  MATLAB Function1/1(v_d) -> Derivative/1, v_d/1
  Demux/1 -> Scope/1, MATLAB Function1/1(e1)
  Demux/2 -> Gain/1, MATLAB Function1/2(e2)
  Demux/3 -> MATLAB Function1/3(e1_dot)
  Demux/4 -> MATLAB Function1/4(e2_dot)
  Demux/5 -> MATLAB Function1/5(gamma)
  Demux/6 -> MATLAB Function1/6(gamma_dot)
  Input/1 -> Demux/1
  Gain/1 -> Scope/3

== system Multiagent_1030_ActorCritic/Subsystem7/RL controller ==
  v_dot : Inport
  eta_r : Inport  Port=2
  eta_r_dot : Inport  Port=3
  v_d : Inport  Port=4
  v : Inport  Port=5
  v_d_dot : Inport  Port=6
  z : Inport  Port=7
  Delay : Delay  DelayLength=1  InitialCondition=[0;0;0]  SampleTime=0.001
  Integrator1 : Integrator  InitialCondition=zeros(15,1)
  Integrator2 : Integrator  InitialCondition=zeros(15,1)
  MATLAB Function : MATLAB Function  TreatAsAtomicUnit=on
  Scope : Scope
  tau : Outport
  wires:
  v/1 -> MATLAB Function/1(v)
  MATLAB Function/1(tau) -> tau/1
  z/1 -> MATLAB Function/7(z)
  v_d_dot/1 -> MATLAB Function/6(v_d_dot)
  v_d/1 -> MATLAB Function/5(v_d)
  eta_r_dot/1 -> MATLAB Function/4(eta_r_dot)
  Integrator1/1 -> MATLAB Function/9(Wa)
  eta_r/1 -> MATLAB Function/3(eta_r)
  Integrator2/1 -> MATLAB Function/8(Wc)
  MATLAB Function/5(Wc_dot) -> Integrator2/1
  MATLAB Function/2(tau_d) -> Scope/1
  MATLAB Function/4(Wa_dot) -> Integrator1/1
  MATLAB Function/3(u) -> Delay/1
  v_dot/1 -> MATLAB Function/2(v_dot)
  Delay/1 -> MATLAB Function/10("u ")

== matlab function Multiagent_1030_ActorCritic/Subsystem1/Dynamics ==
  settings: updateMethod=DISCRETE
  data: t input; tau input; v input; v_dot output; noise output
function [v_dot,noise] = fcn(t,tau,v)
M = [25.8,0,0;0,33.8,1.0948;0,1.0948,2.76];
C = [0,0,-33.8*v(2)-1.0948*v(3);...
    0,0,25.8*v(1);...
    33.8*v(2)+1.0948*v(3),-25.8*v(1),0];
D = [0.7225 + 1.3274*abs(v(1)) + 5.8664*v(1)^2,0,0;...
     0,0.8612+36.2823*abs(v(1)) + 0.805*abs(v(3)),-0.1079 + 0.845*abs(v(1)) + 3.45*abs(v(3));...
     0,-0.1052 - 5.0437*abs(v(1)) - 0.13*abs(v(3)),1.9-0.08*abs(v(2))+0.75*abs(v(3))];

%M = [20,0,0;0,19,0.72;0,0.72,2.7];
% C = [0,0,-19*v(2)-0.72*v(3);0,0,20*v(1);19*v(2)+0.72*v(3),-20*v(1),0];
% 
% D = [0.72+1.3*abs(v(1))+5.8*v(1)^2,0,0;...
% 0,0.86+36*abs(v(2))+3*abs(v(3)),-0.1-2*abs(v(2))+2*abs(v(3));...
% 0,-0.1-5*abs(v(2))+3*abs(v(3)),6+4*abs(v(2))+4*abs(v(3))];

% tau_w=[3-0.2*sin(0.1*t)+0.1*cos(0.02*t)+0.1*rand(1);...
%     - 2.5 + 0.1*cos(0.1*t) + 0.1*sin(0.02*t) + 0.1*rand(1);...
%     3 - 0.2*sin(0.1*t) - 0.1*cos(0.02*t) + 0.1*rand(1)];

if (t < 15)
    flag = 1;
else 
    flag = 0;
end
noise = zeros(3,1);
% noise(1) = (50*sin(25*t) + 65*sin(45*(t-1)) + 45*sin(20*(t-0.5)) + 55*sin(35*(t-1.5)))*flag;
% noise(2) = (20*sin(25*t) + 10*sin(45*(t-1)) + 16*sin(20*(t-0.5)) + 20*sin(35*(t-1.5)))*flag;
% noise(3) = (9*sin(25*t) + 10*sin(45*(t-1)) + 14*sin(20*(t-0.5)) + 30*sin(35*(t-1.5)))*flag;

noise(1) = (10*sin(25*t) + 16*sin(45*(t-1)) + 15*sin(20*(t-0.5)) + 10*sin(35*(t-1.5)))*flag;
noise(2) = (50*sin(25*t) + 50*sin(45*(t-1)) + 40*sin(20*(t-0.5)) + 50*sin(35*(t-1.5)))*flag;
noise(3) = (40*sin(25*t) + 30*sin(45*(t-1)) + 45*sin(20*(t-0.5)) + 40*sin(35*(t-1.5)))*flag/20;

v_dot = -M\C*v-M\D*v+M\(tau  + noise);

== matlab function Multiagent_1030_ActorCritic/Subsystem1/RL controller/Controller ==
  data: tau output; tau_d output; u output; v input; v_dot input; eta_r input; Wa_dot output; Wc_dot output; eta_r_dot input; v_d input; v_d_dot input; z input; Wc input; Wa input; u input; R output; RL parameter
function [tau,tau_d,u,Wa_dot,Wc_dot,R] = fcn(v,v_dot,eta_r,eta_r_dot,v_d,v_d_dot,z,Wc,Wa,u,RL)
%Q=eye(3);R=eye(3);
M = [25.8,0,0;0,33.8,1.0948;0,1.0948,2.76];
%M = [20,0,0;0,19,0.72;0,0.72,2.7];
invM = inv(M);
eta_c = 10;
eta_a1 = 10;
eta_a2 = 20;
nuy = 0.01;
GAMMA = 20; %%khong cap nhat
z2=v-v_d;
z2_dot=v_dot-v_d_dot;
x=[z2;z;eta_r;eta_r_dot];

gradPhi = [2*x(1),0,0;...
             x(2),x(1),0;...
             x(3),0,x(1);...
             0,2*x(2),0;...
             0,x(3),x(2);...
             0,0,2*x(3);...
              2*x(1)*x(7)^2,0,0;...
              0,2*x(2)*x(8)^2,0;...
              0,0,2*x(3)*x(9)^2;...
              2*x(1)*x(4)^2,0,0;...
              0,2*x(2)*x(5)^2,0;...
              0,0,2*x(3)*x(6)^2;...
              2*x(1)*x(10)^2,0,0;...
              0,2*x(2)*x(11)^2,0;...
              0,0,2*x(3)^2*x(12)^2]; 
             %15x3
% Phi = [x(1)^2; x(1)*x(2); x(1)*x(3); x(2)^2; x(2)*x(3); x(3)^2; x(1)^2*x(7)^2; x(2)^2*x(8)^2; ...
%     x(3)^2*x(9)^2; x(1)^2*x(4)^2; x(2)^2*x(5)^2; x(3)^2*x(6)^2;x(1)^2*x(10)^2;x(2)^2*x(11)^2;x(3)^2*x(12)^2];
%J = [cos(eta(3)),-sin(eta(3)),0;sin(eta(3)),cos(eta(3)),0;0,0,1];
% J_dot = [-sin(eta(3))*v(3), -cos(eta(3))*v(3), 0;
%       cos(eta(3))*v(3), -sin(eta(3))*v(3), 0;
%              0, 0, 0];
% C_d = [0,0,-33.8*v(2)-1.0948*v(3);0,0,25.8*v(1);33.8*v(2)+1.0948*v(3),-25.8*v(1),0];
% D_d = [0.7225 + 1.3274*abs(v(1)) + 5.8664*v(1)^2,0,0;...
%      0,0.8612+36.2823*abs(v(1)) + 0.805*abs(v(3)),-0.1079 + 0.845*abs(v(1)) + 3.45*abs(v(3));...
%      0,-0.1052 - 5.0437*abs(v(1)) - 0.13*abs(v(3)),1.9-0.08*abs(v(2))+0.75*abs(v(3))];
C_d = [0,0,-33.8*v_d(2)-1.0948*v_d(3);0,0,25.8*v_d(1);33.8*v_d(2)+1.0948*v_d(3),-25.8*v_d(1),0];
D_d = [0.7225 + 1.3274*abs(v_d(1)) + 5.8664*v_d(1)^2,0,0;...
     0,0.8612+36.2823*abs(v_d(1)) + 0.805*abs(v_d(3)),-0.1079 + 0.845*abs(v_d(1)) + 3.45*abs(v_d(3));...
     0,-0.1052 - 5.0437*abs(v_d(1)) - 0.13*abs(v_d(3)),1.9-0.08*abs(v_d(2))+0.75*abs(v_d(3))];

% C_d = [0,0,-19*v_d(2)-0.72*v_d(3);0,0,20*v_d(1);19*v_d(2)+0.72*v_d(3),-20*v_d(1),0];
% D_d = [0.72+1.3*abs(v_d(1))+5.8*v_d(1)^2,0,0;...
% 0,0.86+36*abs(v_d(2))+3*abs(v_d(3)),-0.1-2*abs(v_d(2))+2*abs(v_d(3));...
% 0,-0.1-5*abs(v_d(2))+3*abs(v_d(3)),6+4*abs(v_d(2))+4*abs(v_d(3))];

% V = Wc'*Phi; 
zigma=gradPhi*z2_dot;
delta_hjb=Wc'*zigma + z2'*z2 + u'*u;
Wc_dot = -eta_c*GAMMA*zigma/(1+nuy*(zigma'*GAMMA*zigma))*delta_hjb;
Wa_dot = -eta_a1/sqrt(1+zigma'*zigma)*gradPhi*(invM*invM')*gradPhi'*(Wa-Wc)*delta_hjb-eta_a2*(Wa-Wc);

tau_d = M*v_d_dot+C_d*v_d+D_d*v_d;

u = -1/2*invM'*gradPhi'*Wa;

if (RL == 0)
    u = [0;0;0];
end

tau = tau_d + u;

Q = [eye(6) zeros(6,6); zeros(6,6) zeros(6)];
R = x'*Q*x + (tau_d + u)'*(tau_d + u);

== matlab function Multiagent_1030_ActorCritic/Subsystem/Dynamics ==
  settings: updateMethod=DISCRETE
  data: t input; tau input; v input; v_dot output
    function v_dot = fcn(t,tau,v)
M = [25.8,0,0;0,33.8,1.0948;0,1.0948,2.76];
C = [0,0,-33.8*v(2)-1.0948*v(3);...
    0,0,25.8*v(1);...
    33.8*v(2)+1.0948*v(3),-25.8*v(1),0];
D = [0.7225 + 1.3274*abs(v(1)) + 5.8664*v(1)^2,0,0;...
     0,0.8612+36.2823*abs(v(1)) + 0.805*abs(v(3)),-0.1079 + 0.845*abs(v(1)) + 3.45*abs(v(3));...
     0,-0.1052 - 5.0437*abs(v(1)) - 0.13*abs(v(3)),1.9-0.08*abs(v(2))+0.75*abs(v(3))];

%M = [20,0,0;0,19,0.72;0,0.72,2.7];
% C = [0,0,-19*v(2)-0.72*v(3);0,0,20*v(1);19*v(2)+0.72*v(3),-20*v(1),0];
% 
% D = [0.72+1.3*abs(v(1))+5.8*v(1)^2,0,0;...
% 0,0.86+36*abs(v(2))+3*abs(v(3)),-0.1-2*abs(v(2))+2*abs(v(3));...
% 0,-0.1-5*abs(v(2))+3*abs(v(3)),6+4*abs(v(2))+4*abs(v(3))];

% tau_w=[3-0.2*sin(0.1*t)+0.1*cos(0.02*t)+0.1*rand(1);...
%     - 2.5 + 0.1*cos(0.1*t) + 0.1*sin(0.02*t) + 0.1*rand(1);...
%     3 - 0.2*sin(0.1*t) - 0.1*cos(0.02*t) + 0.1*rand(1)];

if (t < 15)
    flag = 1;
else 
    flag = 0;
end
noise = zeros(3,1);
% noise(1) = (50*sin(25*t) + 65*sin(45*(t-1)) + 45*sin(20*(t-0.5)) + 55*sin(35*(t-1.5)))*flag;
% noise(2) = (20*sin(25*t) + 10*sin(45*(t-1)) + 16*sin(20*(t-0.5)) + 20*sin(35*(t-1.5)))*flag;
% noise(3) = (9*sin(25*t) + 10*sin(45*(t-1)) + 14*sin(20*(t-0.5)) + 30*sin(35*(t-1.5)))*flag;

noise(1) = (10*sin(25*t) + 16*sin(45*(t-1)) + 15*sin(20*(t-0.5)) + 10*sin(35*(t-1.5)))*flag;
noise(2) = (50*sin(25*t) + 50*sin(45*(t-1)) + 40*sin(20*(t-0.5)) + 50*sin(35*(t-1.5)))*flag;
noise(3) = (40*sin(25*t) + 30*sin(45*(t-1)) + 45*sin(20*(t-0.5)) + 40*sin(35*(t-1.5)))*flag/10;

v_dot = -M\C*v-M\D*v+M\(tau  + noise);

== matlab function Multiagent_1030_ActorCritic/Subsystem1/Kinematics ==
  data: v input; eta_dot output; eta input
function eta_dot = fcn(v,eta)
J = [cos(eta(3)),-sin(eta(3)),0;sin(eta(3)),cos(eta(3)),0;0,0,1];
eta_dot = J*v;

== matlab function Multiagent_1030_ActorCritic/Subsystem1/Kinematics Controller/MATLAB Function4 ==
  data: eta_i_1_dot input; eta_r_dot output; eta_i_1 input; eta_r output
function [eta_r_dot,eta_r] = fcn(eta_i_1_dot,eta_i_1)
d=6;theta=2*pi/3;beta=0;
eta_d=[d*cos(theta);d*sin(theta);beta];
J=[cos(eta_i_1(3)),-sin(eta_i_1(3)),0;
    sin(eta_i_1(3)),cos(eta_i_1(3)),0;
    0,0,1];
J_dot=[-sin(eta_i_1(3))*eta_i_1_dot(3),-cos(eta_i_1(3))*eta_i_1_dot(3),0;
    cos(eta_i_1(3))*eta_i_1_dot(3),-sin(eta_i_1(3))*eta_i_1_dot(3),0;
    0,0,0];
eta_r=eta_i_1 + J*eta_d;
eta_r_dot=eta_i_1_dot + J_dot*eta_d;

== matlab function Multiagent_1030_ActorCritic/Subsystem1/RL controller/MATLAB Function1 ==
  settings: updateMethod=DISCRETE
  data: v input; v_dot input; eta_r input; eta_r_dot input; v_d input; tau output; v_d_dot input; z input; Wc input; Wa input; u input; tau_d output; u output; Wa_dot output; Wc_dot output
function [tau,tau_d,u,Wa_dot,Wc_dot] = fcn(v,v_dot,eta_r,eta_r_dot,v_d,v_d_dot,z,Wc,Wa,u)
%Q=eye(3);R=eye(3);
M = [25.8,0,0;0,33.8,1.0948;0,1.0948,2.76];
%M = [20,0,0;0,19,0.72;0,0.72,2.7];
invM = inv(M);
eta_c = 10;
eta_a1 = 10;
eta_a2 = 20;
nuy = 0.01;
GAMMA = 20; %%khong cap nhat
z2=v-v_d;
z2_dot=v_dot-v_d_dot;
x=[z2;z;eta_r;eta_r_dot];

gradPhi = [2*x(1),0,0;...
             x(2),x(1),0;...
             x(3),0,x(1);...
             0,2*x(2),0;...
             0,x(3),x(2);...
             0,0,2*x(3);...
              2*x(1)*x(7)^2,0,0;...
              0,2*x(2)*x(8)^2,0;...
              0,0,2*x(3)*x(9)^2;...
              2*x(1)*x(4)^2,0,0;...
              0,2*x(2)*x(5)^2,0;...
              0,0,2*x(3)*x(6)^2;...
              2*x(1)*x(10)^2,0,0;...
              0,2*x(2)*x(11)^2,0;...
              0,0,2*x(3)^2*x(12)^2]; 
             %15x3
%Phi = [x(1)^2; x(1)*x(2); x(1)*x(3); x(2)^2; x(2)*x(3); x(3)^2; x(1)^2*x(7)^2; x(2)^2*x(8)^2; ...
%    x(3)^2*x(9)^2; x(1)^2*x(4)^2; x(2)^2*x(5)^2; x(3)^2*x(6)^2;x(1)^2*x(10)^2;x(2)^2*x(11)^2;x(3)^2*x(12)^2];
%J = [cos(eta(3)),-sin(eta(3)),0;sin(eta(3)),cos(eta(3)),0;0,0,1];
% J_dot = [-sin(eta(3))*v(3), -cos(eta(3))*v(3), 0;
%       cos(eta(3))*v(3), -sin(eta(3))*v(3), 0;
%              0, 0, 0];
% C_d = [0,0,-33.8*v(2)-1.0948*v(3);0,0,25.8*v(1);33.8*v(2)+1.0948*v(3),-25.8*v(1),0];
% D_d = [0.7225 + 1.3274*abs(v(1)) + 5.8664*v(1)^2,0,0;...
%      0,0.8612+36.2823*abs(v(1)) + 0.805*abs(v(3)),-0.1079 + 0.845*abs(v(1)) + 3.45*abs(v(3));...
%      0,-0.1052 - 5.0437*abs(v(1)) - 0.13*abs(v(3)),1.9-0.08*abs(v(2))+0.75*abs(v(3))];
C_d = [0,0,-33.8*v_d(2)-1.0948*v_d(3);0,0,25.8*v_d(1);33.8*v_d(2)+1.0948*v_d(3),-25.8*v_d(1),0];
D_d = [0.7225 + 1.3274*abs(v_d(1)) + 5.8664*v_d(1)^2,0,0;...
     0,0.8612+36.2823*abs(v_d(1)) + 0.805*abs(v_d(3)),-0.1079 + 0.845*abs(v_d(1)) + 3.45*abs(v_d(3));...
     0,-0.1052 - 5.0437*abs(v_d(1)) - 0.13*abs(v_d(3)),1.9-0.08*abs(v_d(2))+0.75*abs(v_d(3))];

% C_d = [0,0,-19*v_d(2)-0.72*v_d(3);0,0,20*v_d(1);19*v_d(2)+0.72*v_d(3),-20*v_d(1),0];
% D_d = [0.72+1.3*abs(v_d(1))+5.8*v_d(1)^2,0,0;...
% 0,0.86+36*abs(v_d(2))+3*abs(v_d(3)),-0.1-2*abs(v_d(2))+2*abs(v_d(3));...
% 0,-0.1-5*abs(v_d(2))+3*abs(v_d(3)),6+4*abs(v_d(2))+4*abs(v_d(3))];


zigma=gradPhi*z2_dot;
delta_hjb=Wc'*zigma + z2'*z2 + u'*u;
Wc_dot = -eta_c*GAMMA*zigma/(1+nuy*(zigma'*GAMMA*zigma))*delta_hjb;
Wa_dot = -eta_a1/sqrt(1+zigma'*zigma)*gradPhi*(invM*invM')*gradPhi'*(Wa-Wc)*delta_hjb-eta_a2*(Wa-Wc);

tau_d = M*v_d_dot+C_d*v_d+D_d*v_d;

u = -1/2*invM'*gradPhi'*Wa;

tau = tau_d + u;

== matlab function Multiagent_1030_ActorCritic/MATLAB Function1 ==
  data: input input; v output; w output
function [v,w] = fcn(input)

v = sqrt(input(1)^2+input(2)^2);
w = input(3);
end

== matlab function Multiagent_1030_ActorCritic/MATLAB Function2 ==
  data: input input; v output; w output
function [v,w] = fcn(input)

v = sqrt(input(1)^2+input(2)^2);
w = input(3);
end

== matlab function Multiagent_1030_ActorCritic/MATLAB Function3 ==
  data: input input; v output; w output
function [v,w] = fcn(input)

v = sqrt(input(1)^2+input(2)^2);
w = input(3);
end

== matlab function Multiagent_1030_ActorCritic/MATLAB Function4 ==
  data: input input; v output; w output
function [v,w] = fcn(input)

v = sqrt(input(1)^2+input(2)^2);
w = input(3);
end

== matlab function Multiagent_1030_ActorCritic/Subsystem5/Dynamics ==
  settings: updateMethod=DISCRETE
  data: t input; tau input; v input; v_dot output
    function v_dot = fcn(t,tau,v)
M = [25.8,0,0;0,33.8,1.0948;0,1.0948,2.76];
C = [0,0,-33.8*v(2)-1.0948*v(3);...
    0,0,25.8*v(1);...
    33.8*v(2)+1.0948*v(3),-25.8*v(1),0];
D = [0.7225 + 1.3274*abs(v(1)) + 5.8664*v(1)^2,0,0;...
     0,0.8612+36.2823*abs(v(1)) + 0.805*abs(v(3)),-0.1079 + 0.845*abs(v(1)) + 3.45*abs(v(3));...
     0,-0.1052 - 5.0437*abs(v(1)) - 0.13*abs(v(3)),1.9-0.08*abs(v(2))+0.75*abs(v(3))];

%M = [20,0,0;0,19,0.72;0,0.72,2.7];
% C = [0,0,-19*v(2)-0.72*v(3);0,0,20*v(1);19*v(2)+0.72*v(3),-20*v(1),0];
% 
% D = [0.72+1.3*abs(v(1))+5.8*v(1)^2,0,0;...
% 0,0.86+36*abs(v(2))+3*abs(v(3)),-0.1-2*abs(v(2))+2*abs(v(3));...
% 0,-0.1-5*abs(v(2))+3*abs(v(3)),6+4*abs(v(2))+4*abs(v(3))];

% tau_w=[3-0.2*sin(0.1*t)+0.1*cos(0.02*t)+0.1*rand(1);...
%     - 2.5 + 0.1*cos(0.1*t) + 0.1*sin(0.02*t) + 0.1*rand(1);...
%     3 - 0.2*sin(0.1*t) - 0.1*cos(0.02*t) + 0.1*rand(1)];

if (t < 15)
    flag = 1;
else 
    flag = 0;
end
noise = zeros(3,1);
% noise(1) = (50*sin(25*t) + 65*sin(45*(t-1)) + 45*sin(20*(t-0.5)) + 55*sin(35*(t-1.5)))*flag;
% noise(2) = (20*sin(25*t) + 10*sin(45*(t-1)) + 16*sin(20*(t-0.5)) + 20*sin(35*(t-1.5)))*flag;
% noise(3) = (9*sin(25*t) + 10*sin(45*(t-1)) + 14*sin(20*(t-0.5)) + 30*sin(35*(t-1.5)))*flag;

noise(1) = (10*sin(25*t) + 16*sin(45*(t-1)) + 15*sin(20*(t-0.5)) + 10*sin(35*(t-1.5)))*flag;
noise(2) = (50*sin(25*t) + 50*sin(45*(t-1)) + 40*sin(20*(t-0.5)) + 50*sin(35*(t-1.5)))*flag;
noise(3) = (40*sin(25*t) + 30*sin(45*(t-1)) + 45*sin(20*(t-0.5)) + 40*sin(35*(t-1.5)))*flag/10;

v_dot = -M\C*v-M\D*v+M\(tau  + noise);

== matlab function Multiagent_1030_ActorCritic/Variable Selection ==
  data: eta_0 input; eta_1 input; x_all output; eta_2 input; eta_3 input; eta_4 input; eta_5 input; y_all output; psi_all output; xy_all output
function [x_all,y_all,psi_all,xy_all] = fcn(eta_0, eta_1, eta_2, eta_3, eta_4, eta_5)
x_all=[eta_1(1);eta_2(1);eta_3(1);eta_4(1);eta_5(1);eta_0(1)];
y_all=[eta_1(2);eta_2(2);eta_3(2);eta_4(2);eta_5(2);eta_0(2)];
psi_all=[eta_1(3);eta_2(3);eta_3(3);eta_4(3);eta_5(3);eta_0(3)];
xy_all=[eta_1(1:2);eta_2(1:2);eta_3(1:2);eta_4(1:2);eta_5(1:2)];

% x_all=[eta_1(1);eta_2(1);eta_3(1);eta_0(1)];
% y_all=[eta_1(2);eta_2(2);eta_3(2);eta_0(2)];
% psi_all=[eta_1(3);eta_2(3);eta_3(3);eta_0(3)];
% xy_all=[eta_1(1:2);eta_2(1:2);eta_3(1:2)];

== matlab function Multiagent_1030_ActorCritic/Subsystem5/Kinematics ==
  data: v input; eta_dot output; eta input
function eta_dot = fcn(v,eta)
J = [cos(eta(3)),-sin(eta(3)),0;sin(eta(3)),cos(eta(3)),0;0,0,1];
eta_dot = J*v;

== matlab function Multiagent_1030_ActorCritic/Subsystem5/Kinematics Controller/MATLAB Function1 ==
  data: e1 input; e2 input; e1_dot input; e2_dot input; gamma input; gamma_dot input; eta_r_dot input; e input; v_d output; eta input; z output
function [v_d,z] = fcn(e1,e2,e1_dot,e2_dot,gamma,gamma_dot,eta_r_dot,e,eta)
z=zeros(3,1);
b=zeros(3,1);
for k=1:3
    b(k)=(e2(k)+e(k))/(gamma(k)*(e1(k)-e(k)));
end
for k=1:3
    z(k)=1/2*log((e2(k)+e(k))/(gamma(k)*(e1(k)-e(k))));
end
p=0.5*(1./(e2+e)+1./(e1-e));
q=-0.5*(e2_dot./(e2_dot+e)-e1_dot./(e1_dot-e)-gamma_dot./gamma);
Phi_1=1/p(1)*(-z(1)+q(1)) + eta_r_dot(1);
Phi_2=1/p(2)*(-0.5*z(2)+q(2)) + eta_r_dot(2);
v_d = [Phi_1*cos(eta(3))+Phi_2*sin(eta(3));
      -Phi_1*sin(eta(3))+Phi_2*cos(eta(3));
      1/p(3)*(-z(3)+q(3))+eta_r_dot(3)];

== matlab function Multiagent_1030_ActorCritic/Subsystem5/Kinematics Controller/MATLAB Function4 ==
  data: eta_i_1_dot input; eta_r_dot output; eta_i_1 input; eta_r output
function [eta_r_dot,eta_r] = fcn(eta_i_1_dot,eta_i_1)
d=6;theta=2*pi/3;beta=0;
eta_d=[d*cos(theta);d*sin(theta);beta];
J=[cos(eta_i_1(3)),-sin(eta_i_1(3)),0;
    sin(eta_i_1(3)),cos(eta_i_1(3)),0;
    0,0,1];
J_dot=[-sin(eta_i_1(3))*eta_i_1_dot(3),-cos(eta_i_1(3))*eta_i_1_dot(3),0;
    cos(eta_i_1(3))*eta_i_1_dot(3),-sin(eta_i_1(3))*eta_i_1_dot(3),0;
    0,0,0];
eta_r=eta_i_1 + J*eta_d;
eta_r_dot=eta_i_1_dot + J_dot*eta_d;

== matlab function Multiagent_1030_ActorCritic/Subsystem/Kinematic controller/MATLAB Function1 ==
  data: e1 input; e2 input; e1_dot input; e2_dot input; gamma input; gamma_dot input; eta_r_dot input; e input; v_d output; eta input; z output
function [v_d,z] = fcn(e1,e2,e1_dot,e2_dot,gamma,gamma_dot,eta_r_dot,e,eta)
z=zeros(3,1);
b=zeros(3,1);
for k=1:3
    b(k)=(e2(k)+e(k))/(gamma(k)*(e1(k)-e(k)));
end
for k=1:3
    z(k)=1/2*log((e2(k)+e(k))/(gamma(k)*(e1(k)-e(k))));
end
p=0.5*(1./(e2+e)+1./(e1-e));
q=-0.5*(e2_dot./(e2_dot+e)-e1_dot./(e1_dot-e)-gamma_dot./gamma);
Phi_1=1/p(1)*(-z(1)+q(1)) + eta_r_dot(1);
Phi_2=1/p(2)*(-0.5*z(2)+q(2)) + eta_r_dot(2);
v_d = [Phi_1*cos(eta(3))+Phi_2*sin(eta(3));
      -Phi_1*sin(eta(3))+Phi_2*cos(eta(3));
      1/p(3)*(-z(3)+q(3))+eta_r_dot(3)];

== matlab function Multiagent_1030_ActorCritic/Subsystem5/RL controller/MATLAB Function ==
  settings: updateMethod=DISCRETE
  data: v input; v_dot input; eta_r input; eta_r_dot input; v_d input; tau output; v_d_dot input; z input; Wc input; Wa input; u input; tau_d output; u output; Wa_dot output; Wc_dot output
function [tau,tau_d,u,Wa_dot,Wc_dot] = fcn(v,v_dot,eta_r,eta_r_dot,v_d,v_d_dot,z,Wc,Wa,u)
%Q=eye(3);R=eye(3);
M = [25.8,0,0;0,33.8,1.0948;0,1.0948,2.76];
%M = [20,0,0;0,19,0.72;0,0.72,2.7];
invM = inv(M);
eta_c = 10;
eta_a1 = 10;
eta_a2 = 20;
nuy = 0.01;
GAMMA = 20; %%khong cap nhat
z2=v-v_d;
z2_dot=v_dot-v_d_dot;
x=[z2;z;eta_r;eta_r_dot];

gradPhi = [2*x(1),0,0;...
             x(2),x(1),0;...
             x(3),0,x(1);...
             0,2*x(2),0;...
             0,x(3),x(2);...
             0,0,2*x(3);...
              2*x(1)*x(7)^2,0,0;...
              0,2*x(2)*x(8)^2,0;...
              0,0,2*x(3)*x(9)^2;...
              2*x(1)*x(4)^2,0,0;...
              0,2*x(2)*x(5)^2,0;...
              0,0,2*x(3)*x(6)^2;...
              2*x(1)*x(10)^2,0,0;...
              0,2*x(2)*x(11)^2,0;...
              0,0,2*x(3)^2*x(12)^2]; 
             %15x3
%Phi = [x(1)^2; x(1)*x(2); x(1)*x(3); x(2)^2; x(2)*x(3); x(3)^2; x(1)^2*x(7)^2; x(2)^2*x(8)^2; ...
%    x(3)^2*x(9)^2; x(1)^2*x(4)^2; x(2)^2*x(5)^2; x(3)^2*x(6)^2;x(1)^2*x(10)^2;x(2)^2*x(11)^2;x(3)^2*x(12)^2];
%J = [cos(eta(3)),-sin(eta(3)),0;sin(eta(3)),cos(eta(3)),0;0,0,1];
% J_dot = [-sin(eta(3))*v(3), -cos(eta(3))*v(3), 0;
%       cos(eta(3))*v(3), -sin(eta(3))*v(3), 0;
%              0, 0, 0];
% C_d = [0,0,-33.8*v(2)-1.0948*v(3);0,0,25.8*v(1);33.8*v(2)+1.0948*v(3),-25.8*v(1),0];
% D_d = [0.7225 + 1.3274*abs(v(1)) + 5.8664*v(1)^2,0,0;...
%      0,0.8612+36.2823*abs(v(1)) + 0.805*abs(v(3)),-0.1079 + 0.845*abs(v(1)) + 3.45*abs(v(3));...
%      0,-0.1052 - 5.0437*abs(v(1)) - 0.13*abs(v(3)),1.9-0.08*abs(v(2))+0.75*abs(v(3))];
C_d = [0,0,-33.8*v_d(2)-1.0948*v_d(3);0,0,25.8*v_d(1);33.8*v_d(2)+1.0948*v_d(3),-25.8*v_d(1),0];
D_d = [0.7225 + 1.3274*abs(v_d(1)) + 5.8664*v_d(1)^2,0,0;...
     0,0.8612+36.2823*abs(v_d(1)) + 0.805*abs(v_d(3)),-0.1079 + 0.845*abs(v_d(1)) + 3.45*abs(v_d(3));...
     0,-0.1052 - 5.0437*abs(v_d(1)) - 0.13*abs(v_d(3)),1.9-0.08*abs(v_d(2))+0.75*abs(v_d(3))];

% C_d = [0,0,-19*v_d(2)-0.72*v_d(3);0,0,20*v_d(1);19*v_d(2)+0.72*v_d(3),-20*v_d(1),0];
% D_d = [0.72+1.3*abs(v_d(1))+5.8*v_d(1)^2,0,0;...
% 0,0.86+36*abs(v_d(2))+3*abs(v_d(3)),-0.1-2*abs(v_d(2))+2*abs(v_d(3));...
% 0,-0.1-5*abs(v_d(2))+3*abs(v_d(3)),6+4*abs(v_d(2))+4*abs(v_d(3))];


zigma=gradPhi*z2_dot;
delta_hjb=Wc'*zigma + z2'*z2 + u'*u;
Wc_dot = -eta_c*GAMMA*zigma/(1+nuy*(zigma'*GAMMA*zigma))*delta_hjb;
Wa_dot = -eta_a1/sqrt(1+zigma'*zigma)*gradPhi*(invM*invM')*gradPhi'*(Wa-Wc)*delta_hjb-eta_a2*(Wa-Wc);

tau_d = M*v_d_dot+C_d*v_d+D_d*v_d;

u = -1/2*invM'*gradPhi'*Wa;

tau = tau_d + u;

== matlab function Multiagent_1030_ActorCritic/Subsystem6/Dynamics ==
  settings: updateMethod=DISCRETE
  data: t input; tau input; v input; v_dot output
function v_dot = fcn(t,tau,v)
M = [25.8,0,0;0,33.8,1.0948;0,1.0948,2.76];
C = [0,0,-33.8*v(2)-1.0948*v(3);...
    0,0,25.8*v(1);...
    33.8*v(2)+1.0948*v(3),-25.8*v(1),0];
D = [0.7225 + 1.3274*abs(v(1)) + 5.8664*v(1)^2,0,0;...
     0,0.8612+36.2823*abs(v(1)) + 0.805*abs(v(3)),-0.1079 + 0.845*abs(v(1)) + 3.45*abs(v(3));...
     0,-0.1052 - 5.0437*abs(v(1)) - 0.13*abs(v(3)),1.9-0.08*abs(v(2))+0.75*abs(v(3))];

%M = [20,0,0;0,19,0.72;0,0.72,2.7];
% C = [0,0,-19*v(2)-0.72*v(3);0,0,20*v(1);19*v(2)+0.72*v(3),-20*v(1),0];
% 
% D = [0.72+1.3*abs(v(1))+5.8*v(1)^2,0,0;...
% 0,0.86+36*abs(v(2))+3*abs(v(3)),-0.1-2*abs(v(2))+2*abs(v(3));...
% 0,-0.1-5*abs(v(2))+3*abs(v(3)),6+4*abs(v(2))+4*abs(v(3))];

% tau_w=[3-0.2*sin(0.1*t)+0.1*cos(0.02*t)+0.1*rand(1);...
%     - 2.5 + 0.1*cos(0.1*t) + 0.1*sin(0.02*t) + 0.1*rand(1);...
%     3 - 0.2*sin(0.1*t) - 0.1*cos(0.02*t) + 0.1*rand(1)];

if (t < 15)
    flag = 1;
else 
    flag = 0;
end
noise = zeros(3,1);
% noise(1) = (50*sin(25*t) + 65*sin(45*(t-1)) + 45*sin(20*(t-0.5)) + 55*sin(35*(t-1.5)))*flag;
% noise(2) = (20*sin(25*t) + 10*sin(45*(t-1)) + 16*sin(20*(t-0.5)) + 20*sin(35*(t-1.5)))*flag;
% noise(3) = (9*sin(25*t) + 10*sin(45*(t-1)) + 14*sin(20*(t-0.5)) + 30*sin(35*(t-1.5)))*flag;

noise(1) = (10*sin(25*t) + 16*sin(45*(t-1)) + 15*sin(20*(t-0.5)) + 10*sin(35*(t-1.5)))*flag;
noise(2) = (50*sin(25*t) + 50*sin(45*(t-1)) + 40*sin(20*(t-0.5)) + 50*sin(35*(t-1.5)))*flag;
noise(3) = (40*sin(25*t) + 30*sin(45*(t-1)) + 45*sin(20*(t-0.5)) + 40*sin(35*(t-1.5)))*flag/20;

v_dot = -M\C*v-M\D*v+M\(tau  + noise);

== matlab function Multiagent_1030_ActorCritic/Subsystem6/Kinematics ==
  data: v input; eta_dot output; eta input
function eta_dot = fcn(v,eta)
J = [cos(eta(3)),-sin(eta(3)),0;sin(eta(3)),cos(eta(3)),0;0,0,1];
eta_dot = J*v;

== matlab function Multiagent_1030_ActorCritic/Subsystem6/Kinematics Controller/MATLAB Function1 ==
  data: e1 input; e2 input; e1_dot input; e2_dot input; gamma input; gamma_dot input; eta_r_dot input; e input; v_d output; eta input; z output
function [v_d, z] = fcn(e1, e2, e1_dot, e2_dot, gamma, gamma_dot, eta_r_dot, e, eta)
z=zeros(3,1);
b=zeros(3,1);
for k=1:3
    b(k)=(e2(k)+e(k))/(gamma(k)*(e1(k)-e(k)));
end
for k=1:3
    z(k)=1/2*log((e2(k)+e(k))/(gamma(k)*(e1(k)-e(k))));
end
p=0.5*(1./(e2+e)+1./(e1-e));
q=-0.5*(e2_dot./(e2_dot+e)-e1_dot./(e1_dot-e)-gamma_dot./gamma);
Phi_1=1/p(1)*(-z(1)+q(1)) + eta_r_dot(1);
Phi_2=1/p(2)*(-0.5*z(2)+q(2)) + eta_r_dot(2);
v_d = [Phi_1*cos(eta(3))+Phi_2*sin(eta(3));
      -Phi_1*sin(eta(3))+Phi_2*cos(eta(3));
      1/p(3)*(-z(3)+q(3))+eta_r_dot(3)];

== matlab function Multiagent_1030_ActorCritic/Subsystem6/Kinematics Controller/MATLAB Function4 ==
  data: eta_i_1_dot input; eta_r_dot output; eta_i_1 input; eta_r output
function [eta_r_dot,eta_r] = fcn(eta_i_1_dot,eta_i_1)
d=6;theta=2*pi/3;beta=0;
eta_d=[d*cos(theta);d*sin(theta);beta];
J=[cos(eta_i_1(3)),-sin(eta_i_1(3)),0;
    sin(eta_i_1(3)),cos(eta_i_1(3)),0;
    0,0,1];
J_dot=[-sin(eta_i_1(3))*eta_i_1_dot(3),-cos(eta_i_1(3))*eta_i_1_dot(3),0;
    cos(eta_i_1(3))*eta_i_1_dot(3),-sin(eta_i_1(3))*eta_i_1_dot(3),0;
    0,0,0];
eta_r=eta_i_1 + J*eta_d;
eta_r_dot=eta_i_1_dot + J_dot*eta_d;

== matlab function Multiagent_1030_ActorCritic/Subsystem6/RL controller/MATLAB Function ==
  settings: updateMethod=DISCRETE
  data: v input; v_dot input; eta_r input; eta_r_dot input; v_d input; tau output; v_d_dot input; z input; Wc input; Wa input; u input; tau_d output; u output; Wa_dot output; Wc_dot output
function [tau,tau_d,u,Wa_dot,Wc_dot] = fcn(v,v_dot,eta_r,eta_r_dot,v_d,v_d_dot,z,Wc,Wa,u)
%Q=eye(3);R=eye(3);
M = [25.8,0,0;0,33.8,1.0948;0,1.0948,2.76];
%M = [20,0,0;0,19,0.72;0,0.72,2.7];
invM = inv(M);
eta_c = 10;
eta_a1 = 10;
eta_a2 = 20;
nuy = 0.01;
GAMMA = 20; %%khong cap nhat
z2=v-v_d;
z2_dot=v_dot-v_d_dot;
x=[z2;z;eta_r;eta_r_dot];

gradPhi = [2*x(1),0,0;...
             x(2),x(1),0;...
             x(3),0,x(1);...
             0,2*x(2),0;...
             0,x(3),x(2);...
             0,0,2*x(3);...
              2*x(1)*x(7)^2,0,0;...
              0,2*x(2)*x(8)^2,0;...
              0,0,2*x(3)*x(9)^2;...
              2*x(1)*x(4)^2,0,0;...
              0,2*x(2)*x(5)^2,0;...
              0,0,2*x(3)*x(6)^2;...
              2*x(1)*x(10)^2,0,0;...
              0,2*x(2)*x(11)^2,0;...
              0,0,2*x(3)^2*x(12)^2]; 
             %15x3
%Phi = [x(1)^2; x(1)*x(2); x(1)*x(3); x(2)^2; x(2)*x(3); x(3)^2; x(1)^2*x(7)^2; x(2)^2*x(8)^2; ...
%    x(3)^2*x(9)^2; x(1)^2*x(4)^2; x(2)^2*x(5)^2; x(3)^2*x(6)^2;x(1)^2*x(10)^2;x(2)^2*x(11)^2;x(3)^2*x(12)^2];
%J = [cos(eta(3)),-sin(eta(3)),0;sin(eta(3)),cos(eta(3)),0;0,0,1];
% J_dot = [-sin(eta(3))*v(3), -cos(eta(3))*v(3), 0;
%       cos(eta(3))*v(3), -sin(eta(3))*v(3), 0;
%              0, 0, 0];
% C_d = [0,0,-33.8*v(2)-1.0948*v(3);0,0,25.8*v(1);33.8*v(2)+1.0948*v(3),-25.8*v(1),0];
% D_d = [0.7225 + 1.3274*abs(v(1)) + 5.8664*v(1)^2,0,0;...
%      0,0.8612+36.2823*abs(v(1)) + 0.805*abs(v(3)),-0.1079 + 0.845*abs(v(1)) + 3.45*abs(v(3));...
%      0,-0.1052 - 5.0437*abs(v(1)) - 0.13*abs(v(3)),1.9-0.08*abs(v(2))+0.75*abs(v(3))];
C_d = [0,0,-33.8*v_d(2)-1.0948*v_d(3);0,0,25.8*v_d(1);33.8*v_d(2)+1.0948*v_d(3),-25.8*v_d(1),0];
D_d = [0.7225 + 1.3274*abs(v_d(1)) + 5.8664*v_d(1)^2,0,0;...
     0,0.8612+36.2823*abs(v_d(1)) + 0.805*abs(v_d(3)),-0.1079 + 0.845*abs(v_d(1)) + 3.45*abs(v_d(3));...
     0,-0.1052 - 5.0437*abs(v_d(1)) - 0.13*abs(v_d(3)),1.9-0.08*abs(v_d(2))+0.75*abs(v_d(3))];

% C_d = [0,0,-19*v_d(2)-0.72*v_d(3);0,0,20*v_d(1);19*v_d(2)+0.72*v_d(3),-20*v_d(1),0];
% D_d = [0.72+1.3*abs(v_d(1))+5.8*v_d(1)^2,0,0;...
% 0,0.86+36*abs(v_d(2))+3*abs(v_d(3)),-0.1-2*abs(v_d(2))+2*abs(v_d(3));...
% 0,-0.1-5*abs(v_d(2))+3*abs(v_d(3)),6+4*abs(v_d(2))+4*abs(v_d(3))];


zigma=gradPhi*z2_dot;
delta_hjb=Wc'*zigma + z2'*z2 + u'*u;
Wc_dot = -eta_c*GAMMA*zigma/(1+nuy*(zigma'*GAMMA*zigma))*delta_hjb;
Wa_dot = -eta_a1/sqrt(1+zigma'*zigma)*gradPhi*(invM*invM')*gradPhi'*(Wa-Wc)*delta_hjb-eta_a2*(Wa-Wc);

tau_d = M*v_d_dot+C_d*v_d+D_d*v_d;

u = -1/2*invM'*gradPhi'*Wa;

tau = tau_d + u;
